simulink model "SSB_SC_Receiver_Part_1_2"  (R2022a)
settings: Solver=FixedStepDiscrete  StartTime=0.0  StopTime=inf  RelTol=1e-3
libraries: dspvision x2, matrix_library x2, dspsnks4 x1, dspsigops x1, dspsrcs4 x1
settings Model: Creator=vovan  LastModifiedBy=vovan

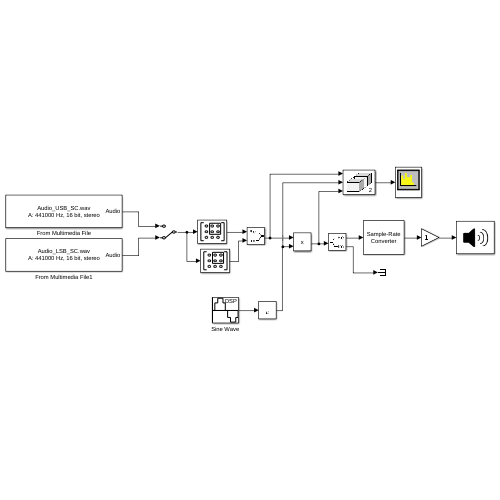
[thumbnail: Simulink's stored preview of the top-level diagram]
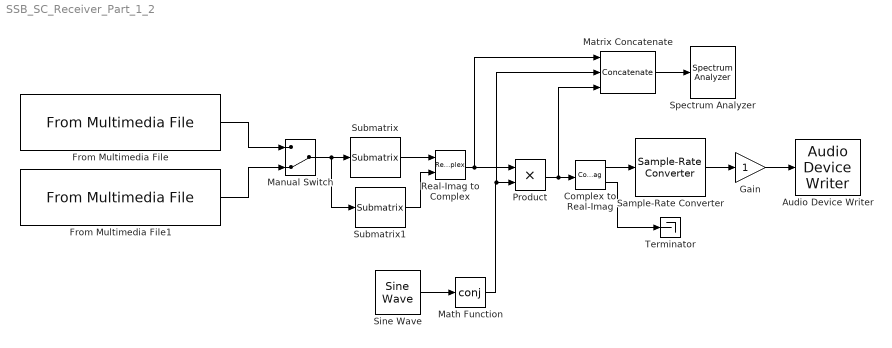
== system SSB_SC_Receiver_Part_1_2 ==
  Audio Device Writer : dspsnks4/Audio Device Writer  Driver=ALSA  Device=Default  InheritSampleRate=on  SampleRate=44100  BitDepth=16-bit integer  BufferSize=4096  NumBuffers=10  DefaultOutputChannelMapping=on  OutputChannelMapping=1:2  OutputNumUnderrunSamples=off  DriverIdx=8  DeviceWarnFlag=''
  Complex to Real-Imag : ComplexToRealImag
  From Multimedia File : dspvision/From Multimedia File  inputFilename=wav/Audio_USB_SC.wav  readRange=[1 Inf]  loop=on  numPlays=inf  outputStreams=Audio only  videoDataType=single  audioDataType=double  inheritSampleTime=on  userDefinedSampleTime=1/30  noAudioOutput=off  isIntensityVideo=off  fourcc=RGB  colorVideoFormat=Separate color signals  outputEOF=off  dataOrg=Column-major  audioFrameSize=10000  computeAudioFrameSize=off  outSamplingMode=Sample based
  From Multimedia File1 : dspvision/From Multimedia File  inputFilename=wav/Audio_LSB_SC.wav  readRange=[1 Inf]  loop=on  numPlays=inf  outputStreams=Audio only  videoDataType=single  audioDataType=double  inheritSampleTime=on  userDefinedSampleTime=1/30  noAudioOutput=off  isIntensityVideo=off  fourcc=RGB  colorVideoFormat=Separate color signals  outputEOF=off  dataOrg=Column-major  audioFrameSize=10000  computeAudioFrameSize=off  outSamplingMode=Sample based
  Gain : Gain
  Manual Switch : ManualSwitch  CurrentSetting=0
  Math Function : Math  Operator=conj
  Matrix Concatenate : Concatenate  NumInputs=3  Mode=Multidimensional array  ConcatenateDimension=2
  Product : Product
  Real-Imag to Complex : RealImagToComplex
  Sample-Rate Converter : dspsigops/Sample-Rate Converter  InputSampleRate=441000  OutputSampleRate=44100  OutputRateTolerance=0  Bandwidth=40e3  StopbandAttenuation=80  SimulateUsing=Code generation
      settings: SourceProductBaseCode=DS
  Sine Wave : dspsrcs4/Sine Wave  Amplitude=1  Frequency=60e3  Phase=0  SampleMode=Discrete  OutComplex=Complex  CompMethod=Trigonometric fcn  TableSize=Speed  SampleTime=1/441000  SamplesPerFrame=10000  ResetState=Restart at time zero  OutputFrames=off  dataType=double  wordLen=16  udDataType=sfix(16)  fracBitsMode=Best precision  numFracBits=15  OutDataTypeStr=double  LastOutDataTypeStr=double
  Spectrum Analyzer : SpectrumAnalyzer
  Submatrix : matrix_library/Submatrix  RowSpan=All rows  RowStartMode=First  RowStartIndex=1  RowEndMode=Last  RowEndIndex=1  ColSpan=Range of columns  ColStartMode=First  ColStartIndex=1  ColEndMode=Index  ColEndIndex=1
      settings: SourceProductBaseCode=SL
  Submatrix1 : matrix_library/Submatrix  RowSpan=All rows  RowStartMode=First  RowStartIndex=1  RowEndMode=Last  RowEndIndex=1  ColSpan=Range of columns  ColStartMode=Last  ColStartIndex=1  ColEndMode=Index  ColEndIndex=1
      settings: SourceProductBaseCode=SL
  Terminator : Terminator
  wires:
  Manual Switch/1 -> Submatrix1/1, Submatrix/1
  Sine Wave/1 -> Math Function/1
  Submatrix/1 -> Real-Imag to Complex/1
  Submatrix1/1 -> Real-Imag to Complex/2
  Real-Imag to Complex/1 -> Matrix Concatenate/1, Product/1
  Complex to Real-Imag/2 -> Terminator/1
  Product/1 -> Matrix Concatenate/3, Complex to Real-Imag/1
  Sample-Rate Converter/1 -> Gain/1
  Complex to Real-Imag/1 -> Sample-Rate Converter/1
  Gain/1 -> Audio Device Writer/1
  Matrix Concatenate/1 -> Spectrum Analyzer/1
  Math Function/1 -> Matrix Concatenate/2, Product/2
  From Multimedia File1/1 -> Manual Switch/2
  From Multimedia File/1 -> Manual Switch/1
